simulink model "exemplo_rastreamento"  (R2019a)
settings: Solver=ode4  StartTime=0.0  StopTime=500  FixedStep=10^-3  RelTol=1e-3  EnableMultiTasking=on
values from neighbouring files (symbols this model uses):
  A = sys.A    [ExampleSS.m]    (also in projeto_Rastereamento.m; simu.m = sys.a)
  B = sys.B    [ExampleSS.m]    (also in projeto_Rastereamento.m; simu.m = sys.b)
  C = sys.C    [ExampleSS.m]    (also in projeto_Rastereamento.m; simu.m = sys.c)
  K = place(A,B,Pd)    [projeto_Rastereamento.m]    (also in simu.m)
  Ki = KK(na(1)+1:end)    [projeto_Rastereamento.m]    (also in simu.m = KK(:,na(1)+1:end))
  Kx = KK(1:na(1))    [projeto_Rastereamento.m]    (also in simu.m = KK(:,1:na(1)))
  N = -1/(C*inv(A-B*K)*B)    [projeto_Rastereamento.m]    (also in simu.m = -1./(C*inv(A-B*K)*B))
settings Model: Creator=Daniel Cruz  LastModifiedBy=Caeta
settings DataIOCC: ReturnWorkspaceOutputs=off
settings OptimizationCC: LifeSpan=inf
settings DebuggingCC: SFUnexpectedBacktrackingDiag=warning  SFNoUnconditionalDefaultTransitionDiag=warning  ArithmeticOperatorsInVariantConditions=warning
settings SFSimCC: SimUseLocalCustomCode=off
settings RTWCC: RTWUseLocalCustomCode=off
settings CodeAppCC: StateflowObjectComments=on
settings GRTTargetCC: TargetLangStandard=C89/C90 (ANSI)  GeneratePreprocessorConditionals=Disable all
settings ConfigComp: CovMetricSettings=dw  CovHtmlReporting=on  CovSaveCumulativeToWorkspaceVar=on  CovSaveSingleToWorkspaceVar=on  CovExternalEMLEnable=off

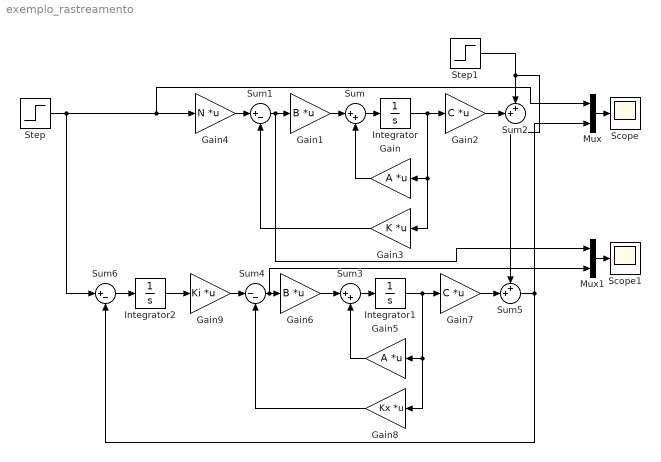
== system exemplo_rastreamento ==
  Gain : Gain  Gain=A  Multiplication=Matrix(K*u)
  Gain1 : Gain  Gain=B  Multiplication=Matrix(K*u)
  Gain2 : Gain  Gain=C  Multiplication=Matrix(K*u)
  Gain3 : Gain  Gain=K  Multiplication=Matrix(K*u)
  Gain4 : Gain  Gain=N  Multiplication=Matrix(K*u)
  Gain5 : Gain  Gain=A  Multiplication=Matrix(K*u)
  Gain6 : Gain  Gain=B  Multiplication=Matrix(K*u)
  Gain7 : Gain  Gain=C  Multiplication=Matrix(K*u)
  Gain8 : Gain  Gain=Kx  Multiplication=Matrix(K*u)
  Gain9 : Gain  Gain=Ki  Multiplication=Matrix(K*u)
  Integrator : Integrator
  Integrator1 : Integrator
  Integrator2 : Integrator
  Mux : Mux  Inputs=2
  Mux1 : Mux  Inputs=2
  Scope : Scope
  Scope1 : Scope
  Step : Step  SampleTime=0
  Step1 : Step  Time=300  SampleTime=0
  Sum : Sum  Inputs=|++
  Sum1 : Sum  Inputs=|+-
  Sum2 : Sum  Inputs=++|
  Sum3 : Sum  Inputs=|++
  Sum4 : Sum  Inputs=|--
  Sum5 : Sum  Inputs=++|
  Sum6 : Sum  Inputs=|+-
  wires:
  Gain1/1 -> Sum/1
  Gain/1 -> Sum/2
  Sum/1 -> Integrator/1
  Integrator/1 -> Gain3/1, Gain/1, Gain2/1
  Gain3/1 -> Sum1/2
  Sum1/1 -> Mux1/1, Gain1/1
  Gain4/1 -> Sum1/1
  Gain2/1 -> Sum2/2
  Gain6/1 -> Sum3/1
  Gain5/1 -> Sum3/2
  Sum3/1 -> Integrator1/1
  Integrator1/1 -> Gain8/1, Gain5/1, Gain7/1
  Gain8/1 -> Sum4/2
  Sum4/1 -> Mux1/2, Gain6/1
  Gain9/1 -> Sum4/1
  Gain7/1 -> Sum5/2
  Step1/1 -> Sum5/1, Sum2/1
  Integrator2/1 -> Gain9/1
  Sum6/1 -> Integrator2/1
  Sum5/1 -> Sum6/2, Mux/2
  Step/1 -> Sum6/1, Mux/1, Gain4/1
  Mux/1 -> Scope/1
  Mux1/1 -> Scope1/1
